simulink model "Flight_simulator"  (R2025b)
settings: Solver=ode4  StartTime=0.0  StopTime=300  FixedStep=0.02  RelTol=1e-3
InitFcn:
  | navion_params;
  | actuator_params;
  | figs0 = findall(0, 'type', 'figure');
  | vis0  = get(0, 'DefaultFigureVisible');
  | set(0, 'DefaultFigureVisible', 'off');
  | evalc('longitudinal_pitch_control; lateral_directional_control;');
  | set(0, 'DefaultFigureVisible', vis0);
  | close(setdiff(findall(0, 'type', 'figure'), figs0));
  | if ~exist('fb_on',   'var'), fb_on   = 1; end
  | if ~exist('gust_on', 'var'), gust_on = 1; end
  | if ~exist('trk_on','var'), trk_on = 1; end
undefined symbols (not defined in the file): A_aug, A_ol_lat, act_on, alt_on, B_lat_open, B_lon_open, F, fb_on, gust_on, h_init, Kh, Ki, Kp, Kphi, Kpsi, Kq, Kv, Kvi, Kxi, Ky, Kzeta, Light, MIL, pos_ail, pos_ele, pos_rud, sens_on, tau_sens, tau_thr, Theta0, trk_on, V0
libraries: aerolibactuator x3, slpidlib x2, aerolibwind2 x1
settings Model: Creator=USER  LastModifiedBy=USER

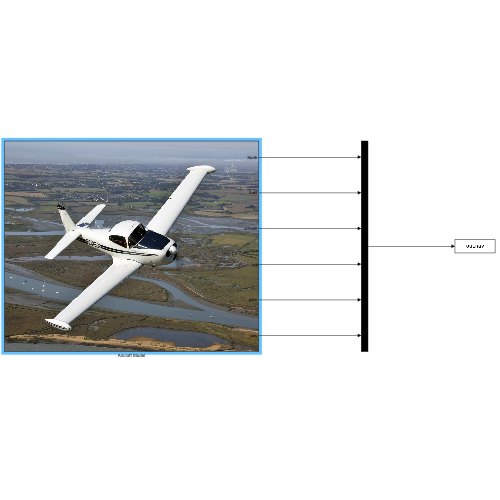
[thumbnail: Simulink's stored preview of the top-level diagram]
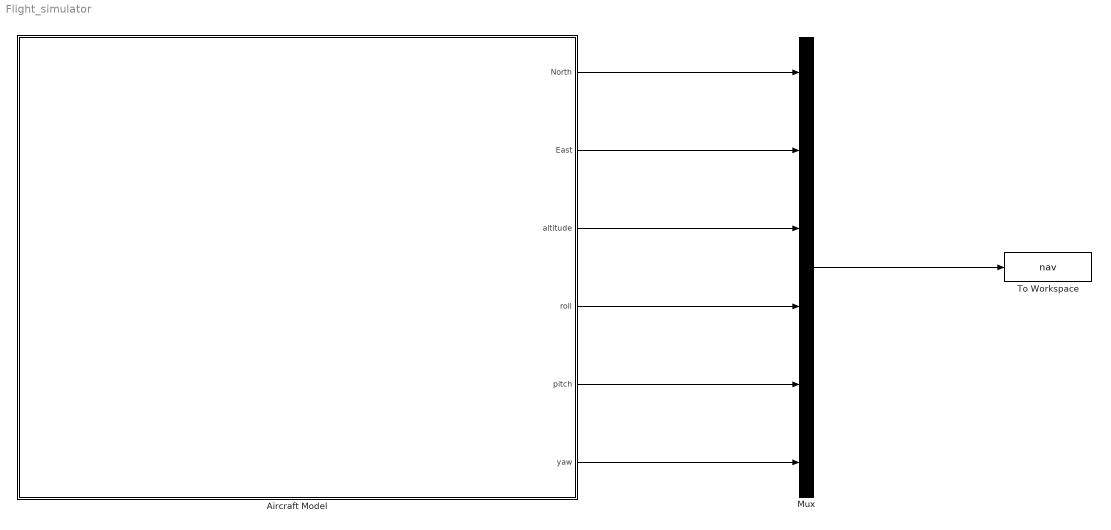
== system Flight_simulator ==
  Aircraft Model : Subsystem
      mask Display: image('img.webp');
  Mux : Mux  Inputs=6
  To Workspace : ToWorkspace  VariableName=nav  SampleTime=-1
  wires:
  Aircraft Model/4(roll) -> Mux/4
  Aircraft Model/5(pitch) -> Mux/5
  Aircraft Model/6(yaw) -> Mux/6
  Aircraft Model/2(East) -> Mux/2
  Aircraft Model/1(North) -> Mux/1
  Aircraft Model/3(altitude) -> Mux/3
  Mux/1 -> To Workspace/1

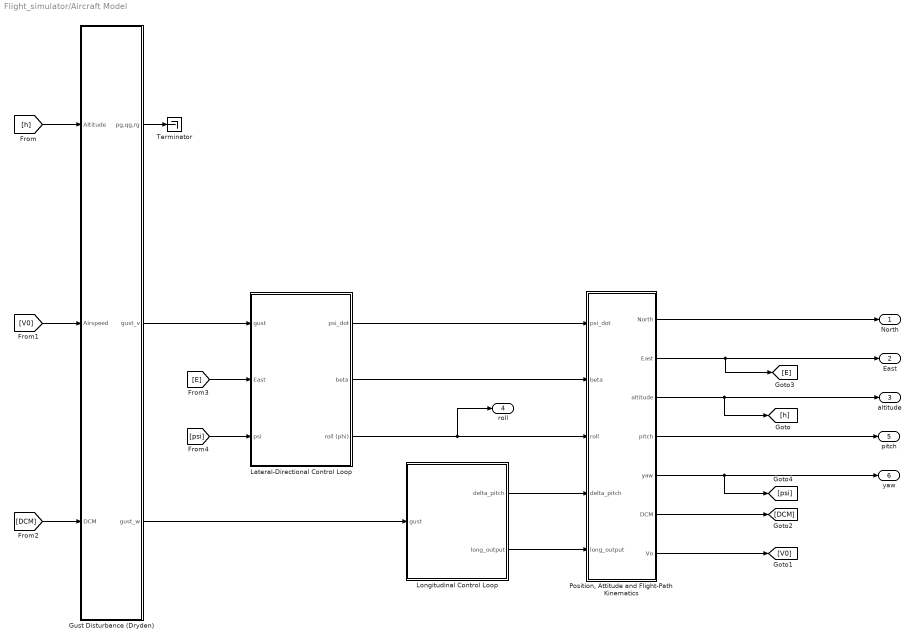
== system Flight_simulator/Aircraft Model ==
  Gust Disturbance (Dryden) : Subsystem
  Lateral-Directional Control Loop : Subsystem
  Longitudinal Control Loop : Subsystem
  "Position, Attitude and Flight-Path Kinematics" : Subsystem
  Terminator : Terminator
  North : Outport
  East : Outport  Port=2
  altitude : Outport  Port=3
  roll : Outport  Port=4
  pitch : Outport  Port=5
  yaw : Outport  Port=6
  wires:
  Gust Disturbance (Dryden)/3(gust_w) -> Longitudinal Control Loop/1(gust)
  [DCM] -> Gust Disturbance (Dryden)/3(DCM)
  [h] -> Gust Disturbance (Dryden)/1(Altitude)
  Lateral-Directional Control Loop/2(beta) -> "Position, Attitude and Flight-Path Kinematics"/2(beta)
  [V0] -> Gust Disturbance (Dryden)/2(Airspeed)
  Lateral-Directional Control Loop/3(roll (phi)) -> roll/1, "Position, Attitude and Flight-Path Kinematics"/3(roll)
  Gust Disturbance (Dryden)/1(pg,qg,rg) -> Terminator/1
  Gust Disturbance (Dryden)/2(gust_v) -> Lateral-Directional Control Loop/1(gust)
  Longitudinal Control Loop/1("delta_pitch ") -> "Position, Attitude and Flight-Path Kinematics"/4(delta_pitch)
  Longitudinal Control Loop/2(long_output) -> "Position, Attitude and Flight-Path Kinematics"/5(long_output)
  Lateral-Directional Control Loop/1(psi_dot) -> "Position, Attitude and Flight-Path Kinematics"/1(psi_dot)
  "Position, Attitude and Flight-Path Kinematics"/2(East) -> [E], East/1
  "Position, Attitude and Flight-Path Kinematics"/1(North) -> North/1
  "Position, Attitude and Flight-Path Kinematics"/3(altitude) -> [h], altitude/1
  "Position, Attitude and Flight-Path Kinematics"/4(pitch) -> pitch/1
  "Position, Attitude and Flight-Path Kinematics"/6(DCM) -> [DCM]
  "Position, Attitude and Flight-Path Kinematics"/7(Vo) -> [V0]
  "Position, Attitude and Flight-Path Kinematics"/5(yaw) -> [psi], yaw/1
  [E] -> Lateral-Directional Control Loop/2(East)
  [psi] -> Lateral-Directional Control Loop/3(psi)

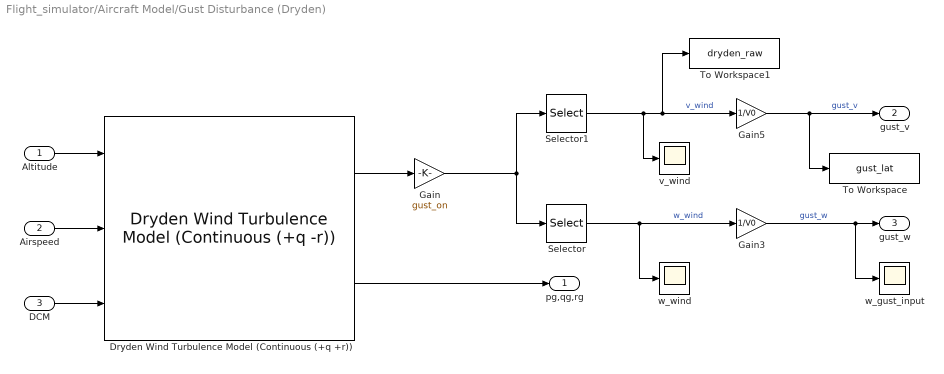
== system Flight_simulator/Aircraft Model/Gust Disturbance (Dryden) ==
  Altitude : Inport
  Airspeed : Inport  Port=2
  DCM : Inport  Port=3
  Dryden Wind Turbulence Model (Continuous (+q +r)) : aerolibwind2/Dryden Wind Turbulence Model  (Continuous (+q -r))  units=Metric (MKS)  spec=MIL-F-8785C  model=Continuous Dryden (+q +r)  W20=15  Wdeg=0  TurbProb=10^-2 - Light  L_high=533.4  Wingspan=10  ts=0.1  Seed=[1030 1031 1032 1033]  T_on=on
      settings: LibrarySourceBlock=|
      | aerolibwind2/Dryden Wind Turbulence Model
      | (Continuous (+q +r))
  Gain : Gain  Gain=gust_on
  Gain3 : Gain  Gain=1/V0
  Gain5 : Gain  Gain=1/V0
  Selector : Selector  InputPortWidth=3  IndexOptions=Index vector (dialog)  Indices=3  OutputSizes=1
  Selector1 : Selector  InputPortWidth=3  IndexOptions=Index vector (dialog)  Indices=2  OutputSizes=1
  To Workspace : ToWorkspace  VariableName=gust_lat  SampleTime=-1
  To Workspace1 : ToWorkspace  VariableName=dryden_raw  SampleTime=-1
  v_wind : Scope
      settings: ActiveDisplayYMinimum=-2.1718299710396272  ActiveDisplayYMaximum=2.2933542366070889  DataLoggingVariableName=ScopeData3
  w_gust_input : Scope
      settings: ActiveDisplayYMinimum=-10.465820831986111  ActiveDisplayYMaximum=10.534179168013885
  w_wind : Scope
      settings: ActiveDisplayYMinimum=-10.465820831986111  ActiveDisplayYMaximum=10.534179168013885  DataLoggingVariableName=ScopeData2
  pg,qg,rg : Outport
  gust_v : Outport  Port=2
  gust_w : Outport  Port=3
  wires:
  Selector1/1 -> v_wind/1, To Workspace1/1, Gain5/1  "v_wind"
  Altitude/1 -> Dryden Wind Turbulence Model (Continuous (+q +r))/1
  Airspeed/1 -> Dryden Wind Turbulence Model (Continuous (+q +r))/2
  Dryden Wind Turbulence Model (Continuous (+q +r))/2 -> pg,qg,rg/1
  DCM/1 -> Dryden Wind Turbulence Model (Continuous (+q +r))/3
  Dryden Wind Turbulence Model (Continuous (+q +r))/1 -> Gain/1
  Selector/1 -> Gain3/1, w_wind/1  "w_wind"
  Gain5/1 -> To Workspace/1, gust_v/1  "gust_v"
  Gain3/1 -> gust_w/1, w_gust_input/1  "gust_w"
  Gain/1 -> Selector/1, Selector1/1

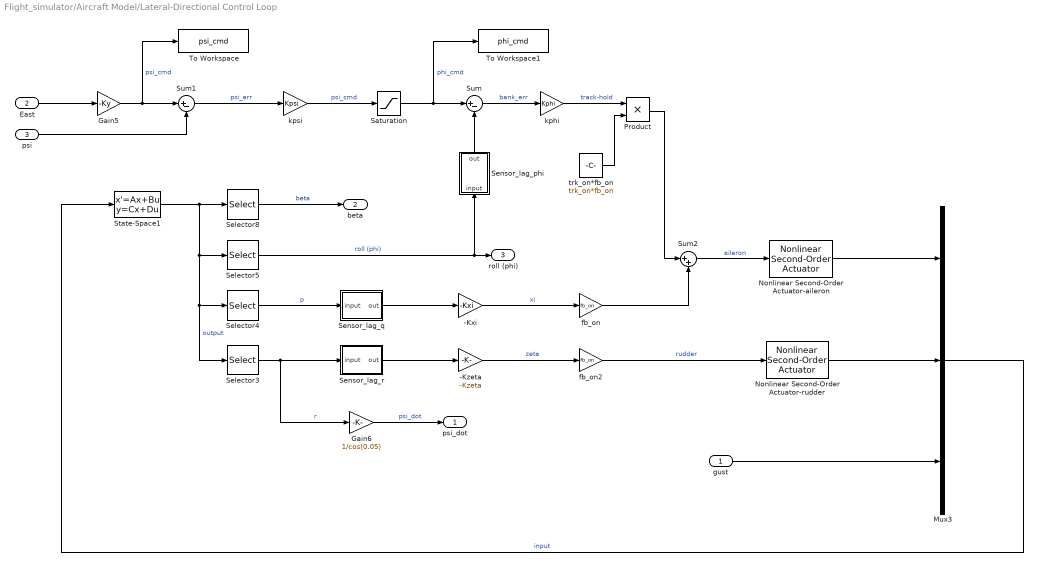
== system Flight_simulator/Aircraft Model/Lateral-Directional Control Loop ==
  gust : Inport
  East : Inport  Port=2
  psi : Inport  Port=3
  -Kxi : Gain  Gain=-Kxi
  -Kzeta : Gain  Gain=-Kzeta
  Gain5 : Gain  Gain=-Ky
  Gain6 : Gain  Gain=1/cos(0.05)
  Mux3 : Mux  Inputs=3
  Nonlinear Second-Order Actuator-aileron : aerolibactuator/Nonlinear Second-Order Actuator  wn_fin=wn_ail  z_fin=zeta_ail  fin_max=pos_ail  fin_min=-pos_ail  fin_maxrate=rate_ail  fin_act_0=0  fin_act_vel=0
  Nonlinear Second-Order Actuator-rudder : aerolibactuator/Nonlinear Second-Order Actuator  wn_fin=wn_rud  z_fin=zeta_rud  fin_max=pos_rud  fin_min=-pos_rud  fin_maxrate=rate_rud  fin_act_0=0  fin_act_vel=0
  Product : Product
  Saturation : Saturate  UpperLimit=0.35  LowerLimit=-0.35
  Selector3 : Selector  InputPortWidth=4  IndexOptions=Index vector (dialog)  Indices=1  OutputSizes=1
  Selector4 : Selector  InputPortWidth=4  IndexOptions=Index vector (dialog)  Indices=3  OutputSizes=1
  Selector5 : Selector  InputPortWidth=4  IndexOptions=Index vector (dialog)  Indices=4  OutputSizes=1
  Selector8 : Selector  InputPortWidth=4  IndexOptions=Index vector (dialog)  Indices=2  OutputSizes=1
  Sensor_lag_phi : Subsystem
  Sensor_lag_q : Subsystem
  Sensor_lag_r : Subsystem
  State-Space1 : StateSpace  A=A_ol_lat  B=B_lat_open  C=eye(4)  D=zeros(4,3)  InitialCondition=0
  Sum : Sum  Inputs=|+-
  Sum1 : Sum  Inputs=|+-
  Sum2 : Sum  Inputs=|++
  To Workspace : ToWorkspace  VariableName=psi_cmd  SampleTime=-1
  To Workspace1 : ToWorkspace  VariableName=phi_cmd  SampleTime=-1
  fb_on : Gain  Gain=fb_on
  fb_on2 : Gain  Gain=fb_on
  kphi : Gain  Gain=Kphi
  kpsi : Gain  Gain=Kpsi
  trk_on*fb_on : Constant  Value=trk_on*fb_on
  psi_dot : Outport
  beta : Outport  Port=2
  roll (phi) : Outport  Port=3
  wires:
  State-Space1/1 -> Selector4/1, Selector3/1, Selector5/1, Selector8/1  "output"
  Selector4/1 -> Sensor_lag_q/1(input)  "p"
  Gain6/1 -> psi_dot/1  "psi_dot"
  Selector5/1 -> roll (phi)/1, Sensor_lag_phi/1(input)  "roll (phi)"
  Selector8/1 -> beta/1  "beta"
  gust/1 -> Mux3/3
  Selector3/1 -> Gain6/1, Sensor_lag_r/1(input)  "r"
  -Kxi/1 -> fb_on/1  "xi"
  -Kzeta/1 -> fb_on2/1  "zeta"
  Mux3/1 -> State-Space1/1  "input"
  fb_on/1 -> Sum2/2
  fb_on2/1 -> Nonlinear Second-Order Actuator-rudder/1  "rudder"
  Gain5/1 -> To Workspace/1, Sum1/1  "psi_cmd"
  Sum1/1 -> kpsi/1  "psi_err"
  kpsi/1 -> Saturation/1  "psi_cmd"
  East/1 -> Gain5/1
  Saturation/1 -> To Workspace1/1, Sum/1  "phi_cmd"
  Sum/1 -> kphi/1  "bank_err"
  kphi/1 -> Product/1  "track-hold"
  Sum2/1 -> Nonlinear Second-Order Actuator-aileron/1  "aileron"
  Product/1 -> Sum2/1
  trk_on*fb_on/1 -> Product/2
  psi/1 -> Sum1/2
  Nonlinear Second-Order Actuator-rudder/1 -> Mux3/2
  Sensor_lag_q/1(out) -> -Kxi/1
  Sensor_lag_r/1(out) -> -Kzeta/1
  Sensor_lag_phi/1(out) -> Sum/2
  Nonlinear Second-Order Actuator-aileron/1 -> Mux3/1

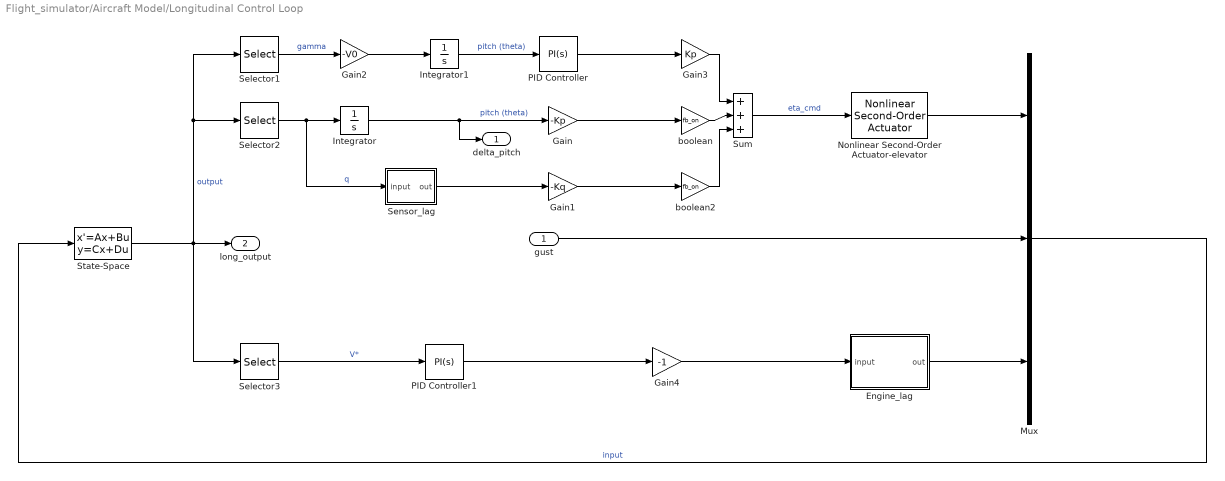
== system Flight_simulator/Aircraft Model/Longitudinal Control Loop ==
  gust : Inport
  Engine_lag : Subsystem  mask{tau=tau_thr, rate_lim=inf, pos_lim=inf}
      mask prompts: tau "Time constant [s]"; rate_lim "Rate limit [rad/s]"; pos_lim "Position limit [rad]"
  Gain : Gain  Gain=-Kp
  Gain1 : Gain  Gain=-Kq
  Gain2 : Gain  Gain=-V0
  Gain3 : Gain  Gain=Kp
  Gain4 : Gain  Gain=-1
  Integrator : Integrator
  Integrator1 : Integrator
  Mux : Mux  Inputs=3
  Nonlinear Second-Order Actuator-elevator : aerolibactuator/Nonlinear Second-Order Actuator  wn_fin=wn_ele  z_fin=zeta_ele  fin_max=pos_ele  fin_min=-pos_ele  fin_maxrate=rate_ele  fin_act_0=0  fin_act_vel=0
  PID Controller : slpidlib/PID Controller  Controller=PI  Form=Parallel  TimeDomain=Continuous-time  UseExternalTs=off  SampleTime=-1  IntegratorMethod=Forward Euler  FilterMethod=Forward Euler  ControllerParametersSource=internal  P=Kh*alt_on  I=Ki*alt_on  UseKiTs=off  D=0  UseExternalDerivativeSource=off  N=100  UseFilter=on  TunerSelectOption=Transfer Function Based (PID Tuner App)  InitialConditionSource=internal  InitialConditionForIntegrator=0  InitialConditionForFilter=0  DifferentiatorICPrevScaledInput=0  ExternalReset=none  TrackingMode=off  Kt=1  LimitOutput=off  SatLimitsSource=internal  UpperSaturationLimit=inf  LowerSaturationLimit=-inf  LinearizeAsGain=on  AntiWindupMode=none  Kb=1  LimitIntegrator=off  UpperIntegratorSaturationLimit=inf  LowerIntegratorSaturationLimit=-inf  POutMin=[]  POutMax=[]  IOutMin=[]  IOutMax=[]  DOutMin=[]  DOutMax=[]  NOutMin=[]  NOutMax=[]  SumOutMin=[]  SumOutMax=[]  SaturationOutMin=[]  SaturationOutMax=[]  PParamMin=[]  PParamMax=[]  IParamMin=[]  IParamMax=[]  DParamMin=[]  DParamMax=[]  NParamMin=[]  NParamMax=[]  KbParamMin=[]  KbParamMax=[]  KtParamMin=[]  KtParamMax=[]  KbOutMin=[]  KbOutMax=[]  KtOutMin=[]  KtOutMax=[]  IntegratorOutMin=[]  IntegratorOutMax=[]  FilterOutMin=[]  FilterOutMax=[]  SumI1OutMin=[]  SumI1OutMax=[]  SumI2OutMin=[]  SumI2OutMax=[]  SumI3OutMin=[]  SumI3OutMax=[]  SumI4OutMin=[]  SumI4OutMax=[]  SumDOutMin=[]  SumDOutMax=[]  DifferentiatorOutMin=[]  DifferentiatorOutMax=[]  FilterDiffOutCoefMin=[]  FilterDiffOutCoefMax=[]  ReciprocalOutMin=[]  ReciprocalOutMax=[]  SumDenOutMin=[]  SumDenOutMax=[]  SumNumOutMin=[]  SumNumOutMax=[]  DivideOutMin=[]  DivideOutMax=[]  UdiffTsProdOutMin=[]  UdiffTsProdOutMax=[]  NTsProdOutMin=[]  NTsProdOutMax=[]  UintegralTsProdOutMin=[]  UintegralTsProdOutMax=[]  UngainTsProdOutMin=[]  UngainTsProdOutMax=[]  ClampingZeroOutDataTypeStr=Inherit: Inherit via back propagation  ClampingZeroOutMin=[]  ClampingZeroOutMax=[]  FilterDenConstantOutDataTypeStr=Inherit: Inherit via back propagation  FilterDenConstantOutMin=[]  FilterDenConstantOutMax=[]  PCopyOutDataTypeStr=Inherit: Inherit via back propagation  PCopyOutMin=[]  PCopyOutMax=[]  NCopyOutDataTypeStr=Inherit: Inherit via back propagation  NCopyOutMin=[]  NCopyOutMax=[]  IntegratorContinuousStateAttributes=''  IntegratorStateMustResolveToSignalObject=off  IntegratorRTWStateStorageClass=Auto  FilterContinuousStateAttributes=''  FilterStateMustResolveToSignalObject=off  FilterRTWStateStorageClass=Auto  ParallelPVariant=InternalParameters  IdealPVariant=Disabled  IVariant=InternalParameters  DVariant=Disabled  IntegratorVariant=Continuous  SatVariant=Disabled  AWVariant=Passthrough  PCopyVariant=Disabled  TRVariant=Disabled  FdbkBlocksVariant=Forward  IdealPFdbkVariant=Disabled  SatFdbkVariant=Disabled  DerivativeFilterVariant=Disabled  NVariant=Disabled  NCopyVariant=Disabled_SignalSpec  FilterICVariant=Disabled  IntegratorICVariant=InternalICs  ExternalResetVariant=Disabled  TRSumVariant=Passthrough  SumFdbkVariant=Disabled  SumVariant=Sum_PI  TsampFilterVariant=InternalTs  TsampNgainVariant=Passthrough  TsampIntegralVariant=Disabled_SignalSpec  ExternalSaturationOutDataTypeStr=Inherit: Same as second input  DerivativeSourceVariant=Disabled  PreIntVariant=InternalPreInt
  PID Controller1 : slpidlib/PID Controller  Controller=PI  Form=Parallel  TimeDomain=Continuous-time  UseExternalTs=off  SampleTime=-1  IntegratorMethod=Forward Euler  FilterMethod=Forward Euler  ControllerParametersSource=internal  P=Kv*alt_on  I=Kvi*alt_on  UseKiTs=off  D=0  UseExternalDerivativeSource=off  N=100  UseFilter=on  TunerSelectOption=Transfer Function Based (PID Tuner App)  InitialConditionSource=internal  InitialConditionForIntegrator=0  InitialConditionForFilter=0  DifferentiatorICPrevScaledInput=0  ExternalReset=none  TrackingMode=off  Kt=1  LimitOutput=off  SatLimitsSource=internal  UpperSaturationLimit=inf  LowerSaturationLimit=-inf  LinearizeAsGain=on  AntiWindupMode=none  Kb=1  LimitIntegrator=off  UpperIntegratorSaturationLimit=inf  LowerIntegratorSaturationLimit=-inf  POutMin=[]  POutMax=[]  IOutMin=[]  IOutMax=[]  DOutMin=[]  DOutMax=[]  NOutMin=[]  NOutMax=[]  SumOutMin=[]  SumOutMax=[]  SaturationOutMin=[]  SaturationOutMax=[]  PParamMin=[]  PParamMax=[]  IParamMin=[]  IParamMax=[]  DParamMin=[]  DParamMax=[]  NParamMin=[]  NParamMax=[]  KbParamMin=[]  KbParamMax=[]  KtParamMin=[]  KtParamMax=[]  KbOutMin=[]  KbOutMax=[]  KtOutMin=[]  KtOutMax=[]  IntegratorOutMin=[]  IntegratorOutMax=[]  FilterOutMin=[]  FilterOutMax=[]  SumI1OutMin=[]  SumI1OutMax=[]  SumI2OutMin=[]  SumI2OutMax=[]  SumI3OutMin=[]  SumI3OutMax=[]  SumI4OutMin=[]  SumI4OutMax=[]  SumDOutMin=[]  SumDOutMax=[]  DifferentiatorOutMin=[]  DifferentiatorOutMax=[]  FilterDiffOutCoefMin=[]  FilterDiffOutCoefMax=[]  ReciprocalOutMin=[]  ReciprocalOutMax=[]  SumDenOutMin=[]  SumDenOutMax=[]  SumNumOutMin=[]  SumNumOutMax=[]  DivideOutMin=[]  DivideOutMax=[]  UdiffTsProdOutMin=[]  UdiffTsProdOutMax=[]  NTsProdOutMin=[]  NTsProdOutMax=[]  UintegralTsProdOutMin=[]  UintegralTsProdOutMax=[]  UngainTsProdOutMin=[]  UngainTsProdOutMax=[]  ClampingZeroOutDataTypeStr=Inherit: Inherit via back propagation  ClampingZeroOutMin=[]  ClampingZeroOutMax=[]  FilterDenConstantOutDataTypeStr=Inherit: Inherit via back propagation  FilterDenConstantOutMin=[]  FilterDenConstantOutMax=[]  PCopyOutDataTypeStr=Inherit: Inherit via back propagation  PCopyOutMin=[]  PCopyOutMax=[]  NCopyOutDataTypeStr=Inherit: Inherit via back propagation  NCopyOutMin=[]  NCopyOutMax=[]  IntegratorContinuousStateAttributes=''  IntegratorStateMustResolveToSignalObject=off  IntegratorRTWStateStorageClass=Auto  FilterContinuousStateAttributes=''  FilterStateMustResolveToSignalObject=off  FilterRTWStateStorageClass=Auto  ParallelPVariant=InternalParameters  IdealPVariant=Disabled  IVariant=InternalParameters  DVariant=Disabled  IntegratorVariant=Continuous  SatVariant=Disabled  AWVariant=Passthrough  PCopyVariant=Disabled  TRVariant=Disabled  FdbkBlocksVariant=Forward  IdealPFdbkVariant=Disabled  SatFdbkVariant=Disabled  DerivativeFilterVariant=Disabled  NVariant=Disabled  NCopyVariant=Disabled_SignalSpec  FilterICVariant=Disabled  IntegratorICVariant=InternalICs  ExternalResetVariant=Disabled  TRSumVariant=Passthrough  SumFdbkVariant=Disabled  SumVariant=Sum_PI  TsampFilterVariant=InternalTs  TsampNgainVariant=Passthrough  TsampIntegralVariant=Disabled_SignalSpec  ExternalSaturationOutDataTypeStr=Inherit: Same as second input  DerivativeSourceVariant=Disabled  PreIntVariant=InternalPreInt
  Selector1 : Selector  InputPortWidth=5  IndexOptions=Index vector (dialog)  Indices=2  OutputSizes=1
  Selector2 : Selector  InputPortWidth=5  IndexOptions=Index vector (dialog)  Indices=4  OutputSizes=1
  Selector3 : Selector  InputPortWidth=5  IndexOptions=Index vector (dialog)  Indices=1  OutputSizes=1
  Sensor_lag : Subsystem
  State-Space : StateSpace  A=A_aug  B=B_lon_open  C=eye(5)  D=zeros(5,3)  InitialCondition=0
  Sum : Sum  Inputs=|+++
  boolean : Gain  Gain=fb_on
  boolean2 : Gain  Gain=fb_on
  "delta_pitch " : Outport
  long_output : Outport  Port=2
  wires:
  Selector2/1 -> Sensor_lag/1(input), Integrator/1  "q"
  Integrator/1 -> Gain/1, "delta_pitch "/1  "pitch (theta)"
  Sum/1 -> Nonlinear Second-Order Actuator-elevator/1  "eta_cmd"
  gust/1 -> Mux/2
  Gain1/1 -> boolean2/1
  Gain/1 -> boolean/1
  Mux/1 -> State-Space/1  "input"
  State-Space/1 -> long_output/1, Selector2/1, Selector1/1, Selector3/1  "output"
  boolean/1 -> Sum/2
  boolean2/1 -> Sum/3
  Selector1/1 -> Gain2/1  "gamma"
  Gain2/1 -> Integrator1/1
  Integrator1/1 -> PID Controller/1  "pitch (theta)"
  Gain3/1 -> Sum/1
  PID Controller/1 -> Gain3/1
  Selector3/1 -> PID Controller1/1  "V*"
  PID Controller1/1 -> Gain4/1
  Gain4/1 -> Engine_lag/1(input)
  Nonlinear Second-Order Actuator-elevator/1 -> Mux/1
  Engine_lag/1(out) -> Mux/3
  Sensor_lag/1(out) -> Gain1/1

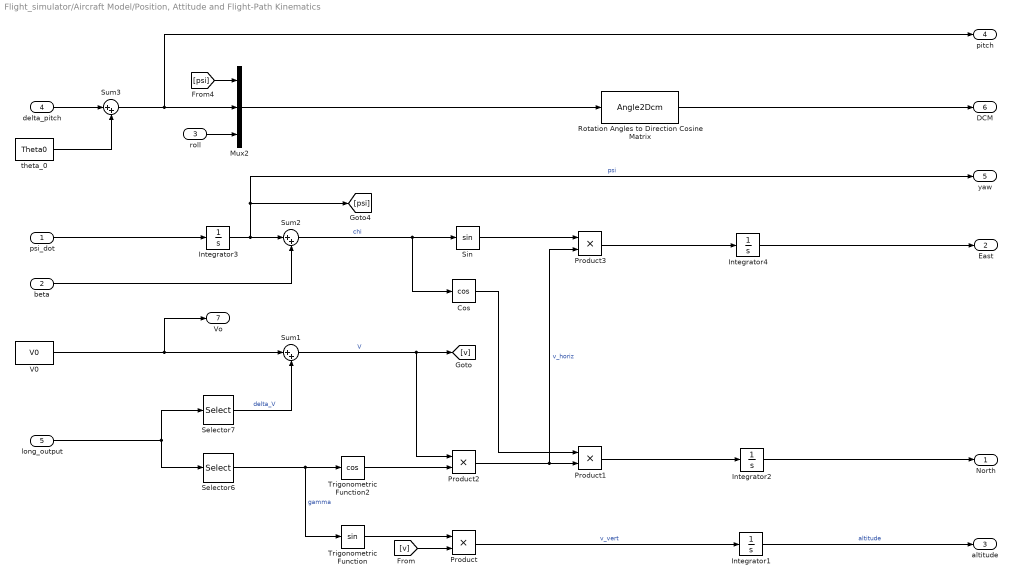
== system Flight_simulator/Aircraft Model/Position, Attitude and Flight-Path Kinematics ==
  psi_dot : Inport
  beta : Inport  Port=2
  roll : Inport  Port=3
  delta_pitch : Inport  Port=4
  long_output : Inport  Port=5
  Cos : Trigonometry  Operator=cos
  Integrator1 : Integrator  InitialCondition=h_init
  Integrator2 : Integrator
  Integrator3 : Integrator
  Integrator4 : Integrator
  Mux2 : Mux  Inputs=3
  Product{,1..3} (4 alike) : Product
  Rotation Angles to Direction Cosine Matrix : Angle2Dcm
      settings: AttributesFormatString=Rotation Order: %<rotationOrder>
  Selector6 : Selector  InputPortWidth=5  IndexOptions=Index vector (dialog)  Indices=2  OutputSizes=1
  Selector7 : Selector  InputPortWidth=5  IndexOptions=Index vector (dialog)  Indices=1  OutputSizes=1
  Sin : Trigonometry
  Sum1 : Sum  Inputs=|++
  Sum2 : Sum  Inputs=|++
  Sum3 : Sum  Inputs=|++
  Trigonometric Function : Trigonometry
  Trigonometric Function2 : Trigonometry  Operator=cos
  V0 : Constant  Value=V0
  theta_0 : Constant  Value=Theta0
  North : Outport
  East : Outport  Port=2
  altitude : Outport  Port=3
  pitch : Outport  Port=4
  yaw : Outport  Port=5
  DCM : Outport  Port=6
  Vo : Outport  Port=7
  wires:
  Integrator2/1 -> North/1
  Sin/1 -> Product3/1
  theta_0/1 -> Sum3/2
  Integrator3/1 -> yaw/1, [psi], Sum2/1  "psi"
  psi_dot/1 -> Integrator3/1
  Selector6/1 -> Trigonometric Function/1, Trigonometric Function2/1  "gamma"
  Sum3/1 -> pitch/1, Mux2/2
  [v] -> Product/2
  Product2/1 -> Product3/2, Product1/2  "v_horiz"
  delta_pitch/1 -> Sum3/1
  [psi] -> Mux2/1
  roll/1 -> Mux2/3
  long_output/1 -> Selector7/1, Selector6/1
  Trigonometric Function/1 -> Product/1
  Mux2/1 -> Rotation Angles to Direction Cosine Matrix/1
  Integrator4/1 -> East/1
  beta/1 -> Sum2/2
  V0/1 -> Vo/1, Sum1/1
  Selector7/1 -> Sum1/2  "delta_V"
  Product/1 -> Integrator1/1  "v_vert"
  Rotation Angles to Direction Cosine Matrix/1 -> DCM/1
  Sum2/1 -> Cos/1, Sin/1  "chi"
  Sum1/1 -> [v], Product2/1  "V"
  Trigonometric Function2/1 -> Product2/2
  Integrator1/1 -> altitude/1  "altitude"
  Cos/1 -> Product1/1
  Product3/1 -> Integrator4/1
  Product1/1 -> Integrator2/1

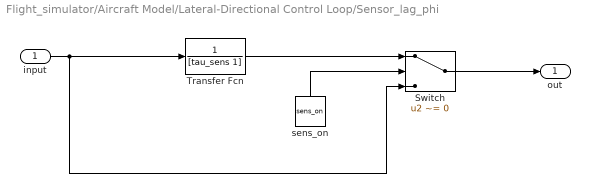
== system Flight_simulator/Aircraft Model/Lateral-Directional Control Loop/Sensor_lag_phi ==
  input : Inport
  Switch : Switch  Criteria=u2 ~= 0  SaturateOnIntegerOverflow=off  InputSameDT=off
  Transfer Fcn : TransferFcn  Denominator=[tau_sens 1]
  sens_on : Constant  Value=sens_on
  out : Outport
  wires:
  Transfer Fcn/1 -> Switch/1
  input/1 -> Transfer Fcn/1, Switch/3
  Switch/1 -> out/1
  sens_on/1 -> Switch/2

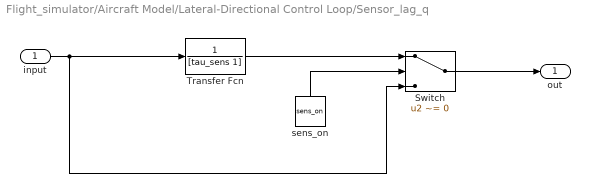
== system Flight_simulator/Aircraft Model/Lateral-Directional Control Loop/Sensor_lag_q ==
  input : Inport
  Switch : Switch  Criteria=u2 ~= 0  SaturateOnIntegerOverflow=off  InputSameDT=off
  Transfer Fcn : TransferFcn  Denominator=[tau_sens 1]
  sens_on : Constant  Value=sens_on
  out : Outport
  wires:
  Transfer Fcn/1 -> Switch/1
  input/1 -> Transfer Fcn/1, Switch/3
  Switch/1 -> out/1
  sens_on/1 -> Switch/2

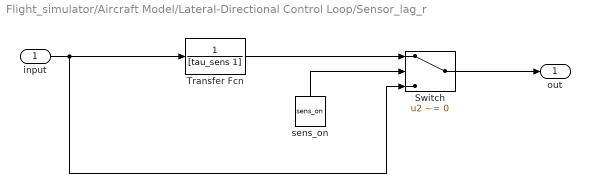
== system Flight_simulator/Aircraft Model/Lateral-Directional Control Loop/Sensor_lag_r ==
  input : Inport
  Switch : Switch  Criteria=u2 ~= 0  SaturateOnIntegerOverflow=off  InputSameDT=off
  Transfer Fcn : TransferFcn  Denominator=[tau_sens 1]
  sens_on : Constant  Value=sens_on
  out : Outport
  wires:
  Transfer Fcn/1 -> Switch/1
  input/1 -> Transfer Fcn/1, Switch/3
  Switch/1 -> out/1
  sens_on/1 -> Switch/2

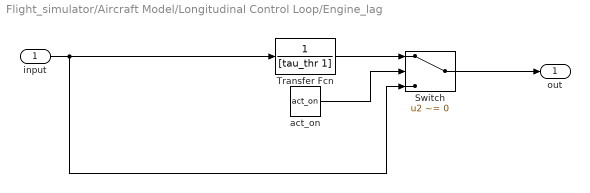
== system Flight_simulator/Aircraft Model/Longitudinal Control Loop/Engine_lag ==
  input : Inport
  Switch : Switch  Criteria=u2 ~= 0  SaturateOnIntegerOverflow=off  InputSameDT=off
  Transfer Fcn : TransferFcn  Denominator=[tau_thr 1]
  act_on : Constant  Value=act_on
  out : Outport
  wires:
  Transfer Fcn/1 -> Switch/1
  input/1 -> Transfer Fcn/1, Switch/3
  Switch/1 -> out/1
  act_on/1 -> Switch/2

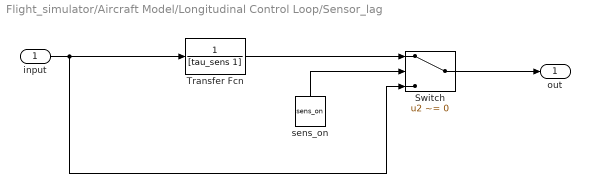
== system Flight_simulator/Aircraft Model/Longitudinal Control Loop/Sensor_lag ==
  input : Inport
  Switch : Switch  Criteria=u2 ~= 0  SaturateOnIntegerOverflow=off  InputSameDT=off
  Transfer Fcn : TransferFcn  Denominator=[tau_sens 1]
  sens_on : Constant  Value=sens_on
  out : Outport
  wires:
  Transfer Fcn/1 -> Switch/1
  input/1 -> Transfer Fcn/1, Switch/3
  Switch/1 -> out/1
  sens_on/1 -> Switch/2
